simulink model "AD9136"  (R2021a)
settings: Solver=FixedStepDiscrete  StartTime=0.0  StopTime=StopTime  FixedStep=1/Fdac  RelTol=1e-3  EnableMultiTasking=on
InitFcn:
  | % Globals
  | NLength = 2^12;
  | Tessitura = 200e6; % Input Frequency
  | L = 1;  % Should match the AD9136 Interpolation
  | Fdac = 2120e6;
  | 
  | % Calculations
  | Fdata = Fdac / L;
  | Samples_per_period = round(1/(Tessitura/Fdata));
  | N_offset_samples = Samples_per_period / 4;
  | 
  | StopTime = NLength / Fdata;
model workspace (MAT data in the model file):
  Res = 16
undefined symbols (not defined in the file or in its folder): tessitura
settings Model: Creator=tmacleod  LastModifiedBy=zhouxxxx
settings SolverCC: AlgebraicLoopSolver=TrustRegion  AutoInsertRateTranBlk=on
settings DataIOCC: LimitDataPoints=on  SaveFormat=Array  ReturnWorkspaceOutputs=off
settings OptimizationCC: LifeSpan=inf
settings DebuggingCC: SolverPrmCheckMsg=warning  SFUnexpectedBacktrackingDiag=warning  SFNoUnconditionalDefaultTransitionDiag=warning  SFExecutionAtInitializationDiag=none  SFMachineParentedDataDiag=warning  ArithmeticOperatorsInVariantConditions=warning
settings HardwareCC: ProdBitPerPointer=32  ProdBitPerSizeT=32  ProdBitPerPtrDiffT=32  ProdLargestAtomicFloat=None  ProdIntDivRoundTo=Undefined  ProdEndianess=Unspecified  ProdWordSize=32  ProdHWDeviceType=32-bit Generic
settings ModelReferenceCC: PropagateSignalLabelsOutOfModel=off
settings SFSimCC: SimUseLocalCustomCode=off  CustomCodeUndefinedFunction=UseInterfaceOnly
settings RTWCC: RTWUseLocalCustomCode=off
settings CodeAppCC: StateflowObjectComments=on
settings GRTTargetCC: TargetLangStandard=C89/C90 (ANSI)
settings ConfigComp: CovMetricSettings=dw  CovSaveCumulativeToWorkspaceVar=on  CovSaveSingleToWorkspaceVar=on  CovExternalEMLEnable=off  CovSFcnEnable=off

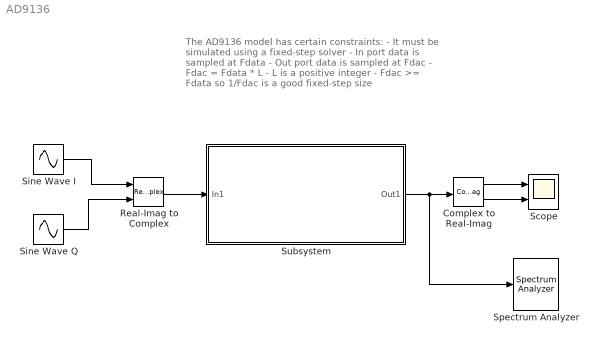
== system AD9136 ==
  note: The AD9136 model has  certain constraints:
      |   - It must be simulated using a fixed-step solver
      |   - In port data is sampled at Fdata
      |   - Out port data is sampled at Fdac
      |   - Fdac = Fdata * L
      |   - L is a positive integer
      |   - Fdac >= Fdata so 1/Fdac is a good fixed-step size
  Complex to Real-Imag : ComplexToRealImag
  Real-Imag to Complex : RealImagToComplex
  Scope : Scope  NumInputPorts=2
  Sine Wave I : Sin  SineType=Sample based  Amplitude=2^(Res-1)  Bias=2^(Res-1)  Frequency=2*pi*tessitura  Samples=Samples_per_period  SampleTime=1/Fdata
  Sine Wave Q : Sin  SineType=Sample based  Amplitude=2^(Res-1)  Bias=2^(Res-1)  Frequency=2*pi*tessitura  Phase=-pi/2  Samples=Samples_per_period  SampleTime=1/Fdata  Offset=N_offset_samples
  Spectrum Analyzer : SpectrumAnalyzer
  Subsystem : Subsystem  mask{L=1, InvSinc=Disabled, Fdata=Fdata}
      mask prompts: L "Interpolation:"; InvSinc "Inverse SINC"
      mask TypeOptions L: 1 | 2 | 4 | 8
      mask TypeOptions InvSinc: Disabled | Enabled
      mask Display: disp('AD9316')
  wires:
  Complex to Real-Imag/1 -> Scope/1
  Complex to Real-Imag/2 -> Scope/2
  Sine Wave I/1 -> Real-Imag to Complex/1
  Sine Wave Q/1 -> Real-Imag to Complex/2
  Subsystem/1(Out1) -> Spectrum Analyzer/1, Complex to Real-Imag/1
  Real-Imag to Complex/1 -> Subsystem/1(In1)

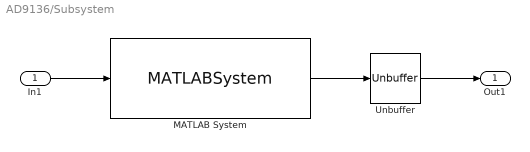
== system AD9136/Subsystem ==
  In1 : Inport
  MATLAB System : MATLABSystem  DialogController=sysobjdialog.BlockDynDialog  System=AD9136_sysobj  Interpolation=1  Fdata=Fdata  InvSinc=Disabled  OutputConfig=Normalized  SimulateUsing=Interpreted execution
      mask Type: AD9136_sysobj
      mask Display:
      | disp('AD9136');
      | port_label('input',1,'in (Code)');
      | port_label('output',1,'out (A)');
  Unbuffer : Unbuffer
  Out1 : Outport
  wires:
  In1/1 -> MATLAB System/1
  MATLAB System/1 -> Unbuffer/1
  Unbuffer/1 -> Out1/1
